simulink model "modelSimple"  (R2025b)
settings: Solver=FixedStepAuto  StartTime=0.0  StopTime=inf  FixedStep=0.01  RelTol=1e-3
model workspace (MAT data in the model file):
  freq = 0.87
settings Model: Creator=marko  LastModifiedBy=Marko
settings DebuggingCC: UnconnectedInputMsg=warning  UnconnectedOutputMsg=warning  UnconnectedLineMsg=warning
settings ModelReferenceCC: EnableRefExpFcnMdlSchedulingChecks=on
settings RTWCC: GPUComputeCapability=3.5  DLArmComputeVersion=19.05

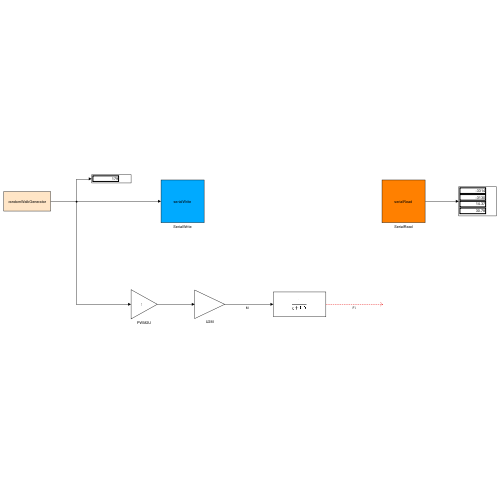
[thumbnail: Simulink's stored preview of the top-level diagram]
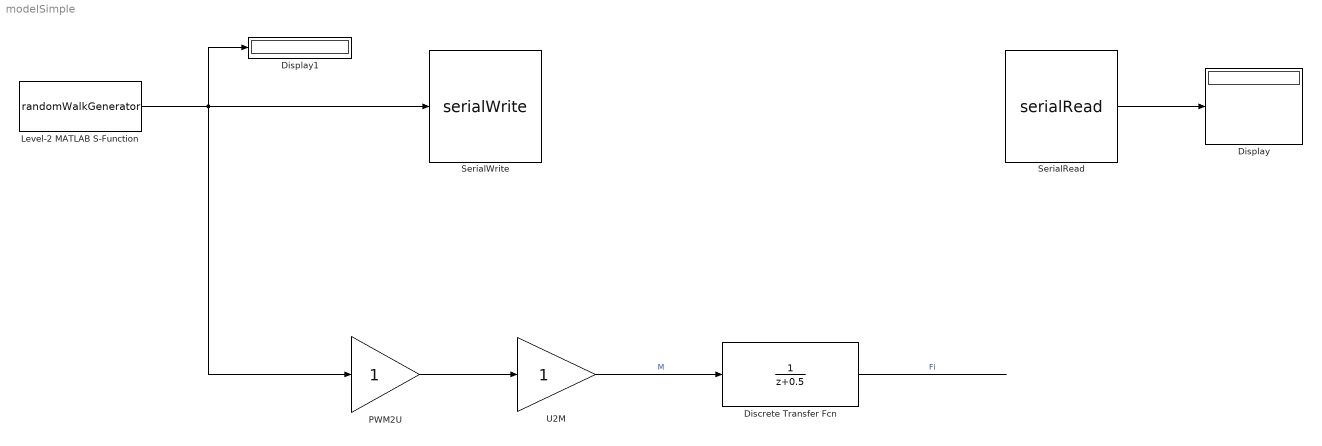
== system modelSimple ==
  Discrete Transfer Fcn : DiscreteTransferFcn
  Display : Display
  Display1 : Display
  Level-2 MATLAB S-Function : M-S-Function  FunctionName=randomWalkGenerator
  PWM2U : Gain
  SerialRead : M-S-Function  FunctionName=serialRead  Parameters='COM4'
  SerialWrite : M-S-Function  FunctionName=serialWrite  Parameters='COM4'
  U2M : Gain
  wires:
  SerialRead/1 -> Display/1
  Level-2 MATLAB S-Function/1 -> PWM2U/1, Display1/1, SerialWrite/1
  Discrete Transfer Fcn/1 -> ?  "Fi"
  PWM2U/1 -> U2M/1
  U2M/1 -> Discrete Transfer Fcn/1  "M"
